simulink model "system_model_simple"  (Simulink 7.4)
settings: Solver=ode15s  StartTime=0.0  StopTime=1  FixedStep=.00001  RelTol=1e-3
values from neighbouring files (symbols this model uses):
  da_coeff = 8.5*10^(-3)    (= 0.0085)    [a2_data_input_examsim1.m]
  dp_coeff = 6*10^(-2)    (= 0.06)    [a2_data_input_examsim1.m]
  dp_freq = 10    [a2_data_input_examsim1.m]
  dp_type = 2    [a2_data_input_examsim1.m]
  dr_coeff = 1    [a2_data_input_examsim1.m]
  dr_h = 0    [a2_data_input_examsim1.m]
  ds_coeff = 1*10^(-3)    (= 0.001)    [a2_data_input_examsim1.m]
  ds_freq = 10000    [a2_data_input_examsim1.m]
  Ga = 3    [a2_data_input_examsim1.m]
  Gd = 1    [a2_data_input_examsim1.m]
  Gf = Gr/(Kd*Gs)    [a3_process_input.m]
  Gr = 1    [a2_data_input_examsim1.m]
  Gs = 1    [a2_data_input_examsim1.m]
libraries: cstblocks x2, simulink x1
settings Model: Creator=s177063  LastModifiedBy=Vittorio
settings DataIOCC: ExternalInput=[t,u]  LimitDataPoints=off  SaveOutput=off
settings DebuggingCC: StrictBusMsg=ErrorLevel1

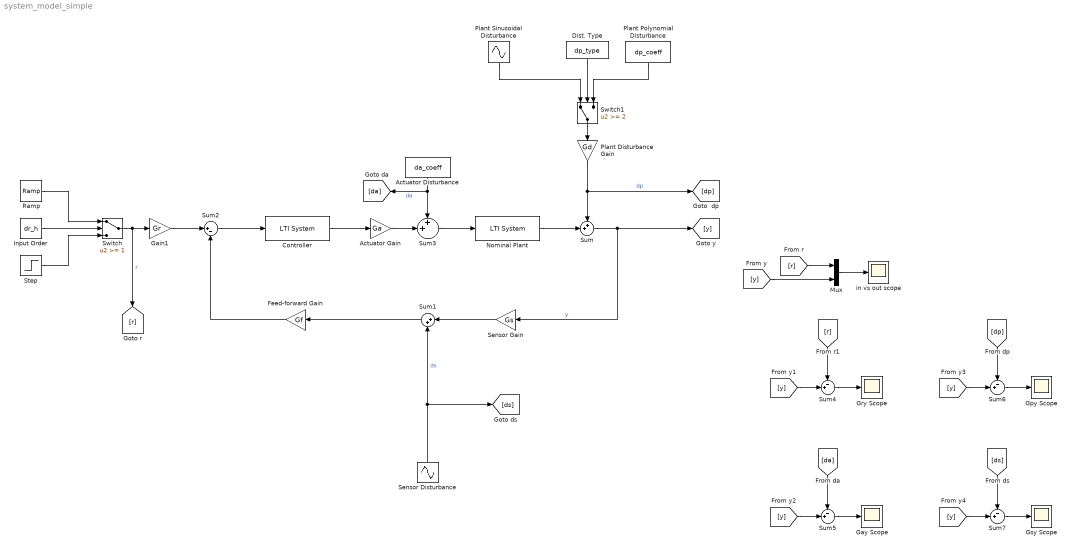
== system system_model_simple ==
  Actuator Disturbance : Constant  Value=da_coeff
  Actuator Gain : Gain  Gain=Ga
  Controller : cstblocks/LTI System  SystemSampleTime=-1  sys=Gcmod  IC=[]
  Dist. Type : Constant  Value=dp_type
  Feed-forward Gain : Gain  Gain=Gf
  Gain1 : Gain  Gain=Gr
  Gay Scope : Scope
      settings: TimeRange=0.5  YMin=0  YMax=2.5  SaveName=ScopeData2  SampleInput=on
  Gpy Scope : Scope
      settings: TimeRange=0.5  YMin=0  YMax=2.5  SaveName=ScopeData4  SampleInput=on
  Gry Scope : Scope
      settings: TimeRange=0.5  YMin=0  YMax=2.5  SampleInput=on
  Gsy Scope : Scope
      settings: TimeRange=0.5  YMin=0  YMax=2.5  SaveName=ScopeData5  SampleInput=on
  Input Order : Constant  Value=dr_h
  Mux : Mux  Inputs=2
  Nominal Plant : cstblocks/LTI System  SystemSampleTime=-1  sys=Gp_nominal  IC=[]
  Plant Disturbance Gain : Gain  Gain=Gd
  Plant Polynomial Disturbance : Constant  Value=dp_coeff
  Plant Sinusoidal Disturbance : Sin  Amplitude=dp_coeff  Bias=0  Frequency=dp_freq  Phase=0  Samples=10  SampleTime=0  Offset=0
  Ramp : simulink/Sources/Ramp  SystemSampleTime=-1  slope=dr_coeff  start=0  X0=0
  Sensor Disturbance : Sin  Amplitude=ds_coeff  Bias=0  Frequency=ds_freq  Phase=0  Samples=10  SampleTime=0  Offset=0
  Sensor Gain : Gain  Gain=Gs
  Step : Step  Time=0  After=dr_coeff  SampleTime=0
  Sum : Sum  Inputs=++|
  Sum1 : Sum  Inputs=|++
  Sum2 : Sum  Inputs=|+-
  Sum3 : Sum  Inputs=++|
  Sum{4..7} (4 alike) : Sum  Inputs=-+|
  Switch : Switch  Threshold=1
  Switch1 : Switch  Threshold=2
  in vs out scope : Scope
      settings: TimeRange=0.5  YMin=1  YMax=2.2  SampleInput=on
  wires:
  Sum/1 -> [y], Sensor Gain/1  "y"
  Controller/1 -> Actuator Gain/1
  Sum3/1 -> Nominal Plant/1
  Gain1/1 -> Sum2/1
  Sum2/1 -> Controller/1
  Sensor Gain/1 -> Sum1/1
  Sum1/1 -> Feed-forward Gain/1
  Feed-forward Gain/1 -> Sum2/2
  Actuator Gain/1 -> Sum3/2
  Nominal Plant/1 -> Sum/2
  Mux/1 -> in vs out scope/1
  Actuator Disturbance/1 -> [da], Sum3/1  "da"
  Input Order/1 -> Switch/2
  Switch/1 -> Gain1/1, [r]  "r"
  Dist. Type/1 -> Switch1/2
  Ramp/1 -> Switch/1
  Step/1 -> Switch/3
  Switch1/1 -> Plant Disturbance Gain/1
  Plant Sinusoidal Disturbance/1 -> Switch1/1
  Plant Polynomial Disturbance/1 -> Switch1/3
  Plant Disturbance Gain/1 -> [dp], Sum/1  "dp"
  Sensor Disturbance/1 -> [ds], Sum1/2  "ds"
  [r] -> Mux/1
  [y] -> Mux/2
  [r] -> Sum4/1
  [y] -> Sum4/2
  Sum4/1 -> Gry Scope/1
  [da] -> Sum5/1
  [y] -> Sum5/2
  Sum5/1 -> Gay Scope/1
  [dp] -> Sum6/1
  [y] -> Sum6/2
  Sum6/1 -> Gpy Scope/1
  [ds] -> Sum7/1
  [y] -> Sum7/2
  Sum7/1 -> Gsy Scope/1
